simulink model "practice_0"  (R2025a)
settings: Solver=VariableStepAuto  StartTime=0.0  StopTime=10.0  RelTol=1e-3
settings Model: Creator=vishwanth  LastModifiedBy=vishwanth

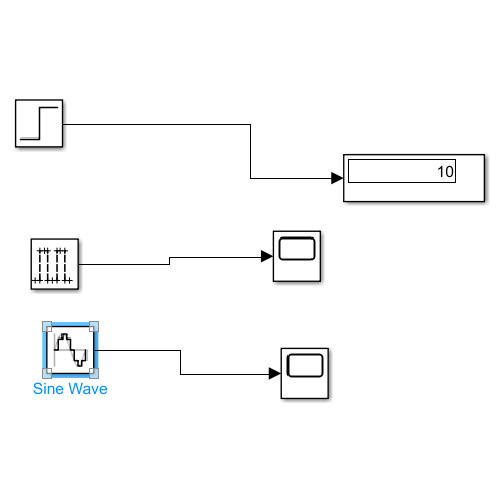
[thumbnail: Simulink's stored preview of the top-level diagram]
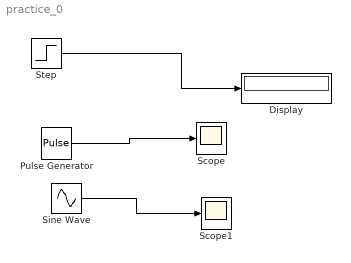
== system practice_0 ==
  Display : Display
  Pulse Generator : DiscretePulseGenerator  Period=10  PulseWidth=2
  Scope : Scope
      settings: ActiveDisplayYMinimum=-0.1435613682092555  ActiveDisplayYMaximum=1.2345636317907445
  Scope1 : Scope
      settings: ActiveDisplayYMinimum=-0.177303940832495  ActiveDisplayYMaximum=1.2697273091675052
  Sine Wave : Sin  Frequency=2  Phase=1  SampleTime=0.5
  Step : Step  Time=2  After=10  SampleTime=0
  wires:
  Step/1 -> Display/1
  Pulse Generator/1 -> Scope/1
  Sine Wave/1 -> Scope1/1
